simulink model "OBSDTC2DOF"  (R2023a)
settings: Solver=VariableStepAuto  StartTime=0.0  StopTime=100  RelTol=1e-3
libraries: cstblocks x4, simulink x2
settings Model: Creator=jprmj  LastModifiedBy=juan
settings OptimizationCC: ReuseModelBlockBuffer=off

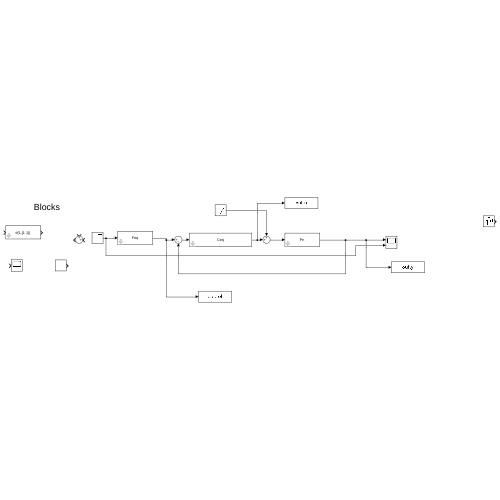
[thumbnail: Simulink's stored preview of the top-level diagram]
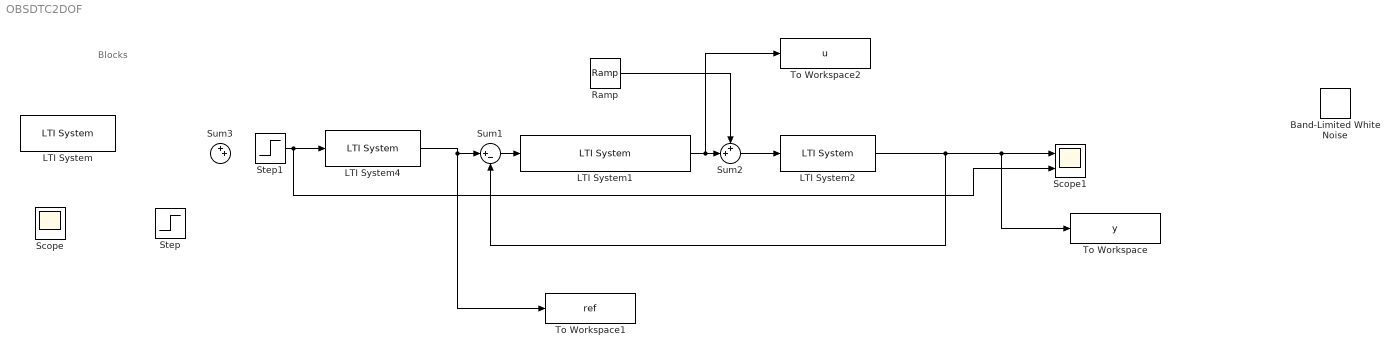
== system OBSDTC2DOF ==
  note: Blocks
  Band-Limited White Noise : simulink/Sources/Band-Limited White Noise  Cov=[0.1]  Ts=0.1  seed=[23341]
  LTI System : cstblocks/LTI System  sys=tf(1,[1 1])  IC=[]
  LTI System1 : cstblocks/LTI System  sys=Ceq  IC=[]
  LTI System2 : cstblocks/LTI System  sys=Pn  IC=[]
  LTI System4 : cstblocks/LTI System  sys=Feq  IC=[]
  Ramp : simulink/Sources/Ramp  slope=0.1  start=65  InitialOutput=0
  Scope : Scope
  Scope1 : Scope  NumInputPorts=2
  Step : Step  SampleTime=0
  Step1 : Step  SampleTime=0
  Sum1 : Sum  Inputs=|+-
  Sum2 : Sum  Inputs=++|
  Sum3 : Sum  Inputs=++|
  To Workspace : ToWorkspace  VariableName=y  SaveFormat=Timeseries  SampleTime=-1
  To Workspace1 : ToWorkspace  VariableName=ref  SaveFormat=Timeseries  SampleTime=-1
  To Workspace2 : ToWorkspace  VariableName=u  SaveFormat=Timeseries  SampleTime=-1
  wires:
  Sum2/1 -> LTI System2/1
  LTI System1/1 -> To Workspace2/1, Sum2/2
  LTI System2/1 -> Sum1/2, To Workspace/1, Scope1/1
  LTI System4/1 -> To Workspace1/1, Sum1/1
  Sum1/1 -> LTI System1/1
  Step1/1 -> Scope1/2, LTI System4/1
  Ramp/1 -> Sum2/1
